simulink model "SL_MOTION"  (R2018b)
settings: Solver=VariableStepAuto  StartTime=0.0  StopTime=10.0  RelTol=1e-3
undefined symbols (not defined in the file): a, v_init, y_init
settings Model: Creator=student  LastModifiedBy=student

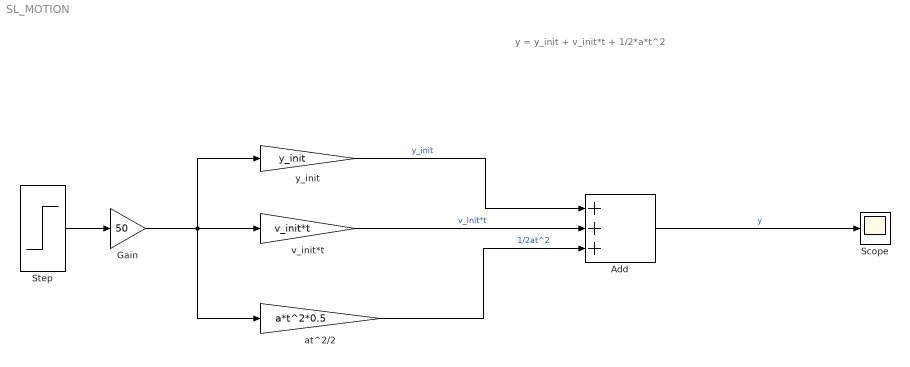
== system SL_MOTION ==
  note: y = y_init + v_init*t + 1/2*a*t^2
  Add : Sum  Inputs=+|+|+
  Gain : Gain  Gain=50
  Scope : Scope
  Step : Step  Time=5  SampleTime=0
  at^2/2 : Gain  Gain=a*t^2*0.5
  v_init*t : Gain  Gain=v_init*t
  y_init : Gain  Gain=y_init
  wires:
  Add/1 -> Scope/1  "y"
  y_init/1 -> Add/1  "y_init"
  v_init*t/1 -> Add/2  "v_init*t"
  at^2/2/1 -> Add/3  "1/2at^2"
  Step/1 -> Gain/1
  Gain/1 -> y_init/1, v_init*t/1, at^2/2/1
